simulink model "ncd_pol_1"  (Simulink 4.00)
settings: Solver=ode45  StartTime=0.0  StopTime=30  RelTol=1e-3
values from neighbouring files (symbols this model uses):
  C = my_sys1.c    [ncd_estim1.m]    (also in ncd_estim_1.mat = [0 0 0 0 0 0.4608]; ncd_kalm1.m; ncd_kalm2.m; ncd_kalm_1.mat = [0 0 0 0 0 0.4608])
  k1 = K(1)    [ncd_estim1.m]    (also in ncd_estim_1.mat = 10.519155687; ncd_kalm1.m; ncd_kalm2.m; ncd_kalm_1.mat = 10.3892921825)
  k2 = K(2)    [ncd_estim1.m]    (also in ncd_estim_1.mat = 9.58454475284; ncd_kalm1.m; ncd_kalm2.m; ncd_kalm_1.mat = 9.59846223426)
  k3 = K(3)    [ncd_estim1.m]    (also in ncd_estim_1.mat = 14.1110774958; ncd_kalm1.m; ncd_kalm2.m; ncd_kalm_1.mat = 13.0219696524)
  k4 = K(4)    [ncd_estim1.m]    (also in ncd_estim_1.mat = 11.3050009574; ncd_kalm1.m; ncd_kalm2.m; ncd_kalm_1.mat = 12.2283669119)
  k5 = K(5)    [ncd_estim1.m]    (also in ncd_estim_1.mat = 6.76215265856; ncd_kalm1.m; ncd_kalm2.m; ncd_kalm_1.mat = 6.58515605602)
  k6 = K(6)    [ncd_estim1.m]    (also in ncd_estim_1.mat = 4.54136711963; ncd_kalm1.m; ncd_kalm2.m; ncd_kalm_1.mat = 4.97835875679)
libraries: cstblocks x1
settings Model: LastModifiedBy=Administrator  BlockReductionOpt=off

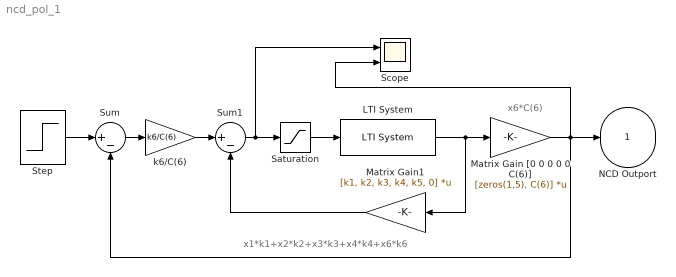
== system ncd_pol_1 ==
  note: x6*C(6)
  note: x1*k1+x2*k2+x3*k3+x4*k4+x6*k6
  LTI System : cstblocks/LTI System  sys=my_sys_n  IC=0
  Matrix Gain [0 0 0 0 0 C(6)] : Gain  Gain=[zeros(1,5), C(6)]  Multiplication=Matrix(K*u)  SaturateOnIntegerOverflow=on
  Matrix Gain1 : Gain  Orientation=left  Gain=[k1, k2, k3, k4, k5, 0]  Multiplication=Matrix(K*u)  SaturateOnIntegerOverflow=on
  Saturation : Saturate  UpperLimit=20  LowerLimit=-20  LinearizeAsGain=on
  Scope : Scope  NumInputPorts=2
      settings: TimeRange=auto  YMin=-5~-5  YMax=5~5  SaveToWorkspace=off  SaveName=ScopeData  LimitDataPoints=on  MaxDataPoints=5000
  Step : Step  Time=0  Before=0  After=1  SampleTime=0
  Sum : Sum  Inputs=|+-  SaturateOnIntegerOverflow=on
  Sum1 : Sum  Inputs=|+-  SaturateOnIntegerOverflow=on
  k6/C(6) : Gain  Gain=k6/C(6)  Multiplication=Element-wise(K.*u)  SaturateOnIntegerOverflow=on
  NCD Outport : Outport  Port=1  InitialOutput=0
      settings: OpenFcn=optblock
      mask Type: NCD Outport
      mask Display:
      | plot([0:10],[-.5 1.5 .6 1.3 .8 1.1 .95 1.02 .99 1 1]);
      | disp('\n\n NCD\n OutPort 1');
  wires:
  LTI System/1 -> Matrix Gain [0 0 0 0 0 C(6)]/1, Matrix Gain1/1
  Matrix Gain [0 0 0 0 0 C(6)]/1 -> NCD Outport/1, Scope/2, Sum/2
  Step/1 -> Sum/1
  Sum/1 -> k6/C(6)/1
  k6/C(6)/1 -> Sum1/1
  Sum1/1 -> Scope/1, Saturation/1
  Matrix Gain1/1 -> Sum1/2
  Saturation/1 -> LTI System/1
